simulink model "CW"  (R2021b)
settings: Solver=VariableStepAuto  StartTime=0.0  StopTime=25  RelTol=1e-3
libraries: simulink x1
settings Model: Creator=piyus  LastModifiedBy=piyus

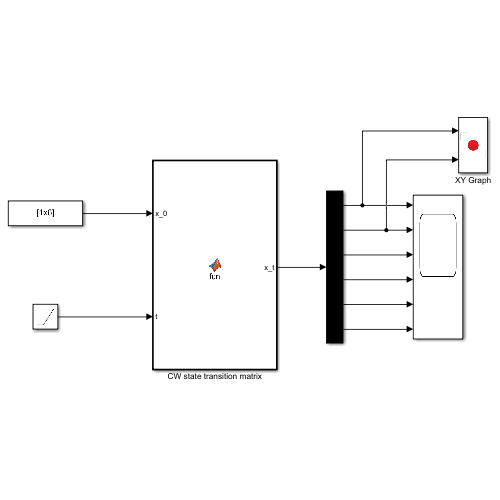
[thumbnail: Simulink's stored preview of the top-level diagram]
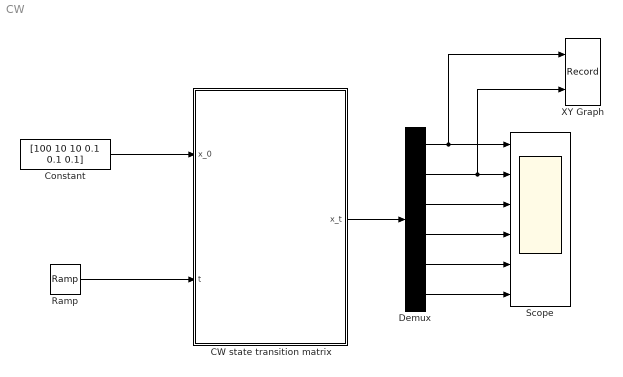
== system CW ==
  CW state transition matrix : MATLAB Function  TreatAsAtomicUnit=on
  Constant : Constant  Value=[100 10 10 0.1 0.1 0.1]
  Demux : Demux  Outputs=6
  Ramp : simulink/Sources/Ramp  slope=1  start=0  InitialOutput=0
  Scope : Scope  NumInputPorts=6
  XY Graph : Record  FileSettingsInternal="{\"entries\":[{\"content\":{\"excelSettings\":{\"content\":{},\"type\":\"Streamout.ExcelSettings\"}},\"type\":\"Streamout.FileSettingStorage\",\"uuid\":\"df4b2df6-b4f8-4ff2-94f6-181a331ec71c\"}],\"packageUris\":[\"http://schema.mathworks.com/mf0/streamout_blocks/R2020a\"],\"version\":\"1.0\"}"  Layout=[1 1]  SignalsInternal="{\"entries\":[{\"content\":{\"signals\":[{\"content\":{\"blockPath\":[\"CW/XY Graph\"],\"channel\":[],\"dimensions\":[1,1],\"domain\":\"CW/XY Graph\",\"lineColor\":\"#a2142f\",\"plots\":[1],\"port\":1,\"sid\":[\"\"],\"signalID\":52,\"signalName\":\"Demux:1\"},\"type\":\"RecordBlkView.Signal\",\"uuid\":\"b5b807f7-e682-429c-8dfe-6263383b7aa0\"},{\"content\":{\"blockPath\":[\"CW/XY Graph\"],\"channel\":[],\"dimensions\":[1,1],\"domain\":\"CW/XY Graph\",\"lineColor\":\"#139fff\",\"plots\":[1],\"port\":2,\"sid\":[\"\"],\"signalID\":56,\"signalName\":\"Demux:2\"},\"type\":\"RecordBlkView.Signal\",\"uuid\":\"4b53b47a-d001-41b6-93cf-bed5810c0147\"}]},\"type\":\"RecordBlkView.InputSignals\",\"uuid\":\"c3eafe66-5bf5-4265-b92d-f2ec2c750c21\"}],\"packageUris\":[\"http://schema.mathworks.com/mf0/streamout_blocks/R2020a\"],\"version\":\"1.0\"}"  VisualizationBindings="{\"xyplotplugin\":{\"info\":[{\"series\":[{\"bindingParametersList\":[{\"parameter\":\"X-Axis\",\"signalID\":52,\"signalName\":\"Demux:1\"},{\"parameter\":\"Y-Axis\",\"signalID\":56,\"signalName\":\"Demux:2\"}],\"seriesID\":54562}],\"subplotID\":1}]}}"  CompatibilityTag=XY
  wires:
  Constant/1 -> CW state transition matrix/1(x_0)
  CW state transition matrix/1(x_t) -> Demux/1
  Ramp/1 -> CW state transition matrix/2(t)
  Demux/1 -> XY Graph/1, Scope/1
  Demux/2 -> XY Graph/2, Scope/2
  Demux/3 -> Scope/3
  Demux/4 -> Scope/4
  Demux/5 -> Scope/5
  Demux/6 -> Scope/6

== matlab function CW/CW state transition matrix ==
  data: x_0 input; x_t output; t input
function x_t = fcn(x_0, t)
R = 6.317e6;
alt = 10e3;
G = 6.67e-11;
M = 5.972e24;
myu = G*M;
w = (myu/(R+alt)^3)^(1/2);
x_t = [(4-3*cos(w*t)), 0, 0, (1/w)*sin(w*t), (2/w)*(1 - cos(w*t)), 0; 6*(sin(w*t)-w*t), 1, 0, (-2/w)*(1 - cos(w*t)), (1/w)*(4*sin(w*t) - 3*w*t), 0; 0, 0, cos(w*t), 0, 0, (1/w)*sin(w*t); 3*w*sin(w*t), 0, 0, cos(w*t), 2*sin(w*t), 0; -6*w*(1-cos(w*t)), 0, 0, -2*sin(w*t), (4*cos(w*t) - 3), 0; 0, 0, -w*sin(w*t), 0, 0, cos(w*t)]*x_0;
